simulink model "CartENDI18a"  (R2018a)
settings: Solver=VariableStepAuto  StartTime=0.0  StopTime=Tsim*Nruns  RelTol=1e-3
values from neighbouring files (symbols this model uses):
  delta_t = 0.01    [init.m]
  x0 = [-10; 10; pi/2; 0; 0]    [init.m]    (also in myFindInitState.m = findstates(sys, dataset))
undefined symbols (not defined in the file or in its folder): pars, theta_star
libraries: simulink x1
settings Model: Creator=Osinenko  LastModifiedBy=pavel
settings SFSimCC: SimUseLocalCustomCode=on
settings RTWCC: RTWUseLocalCustomCode=on

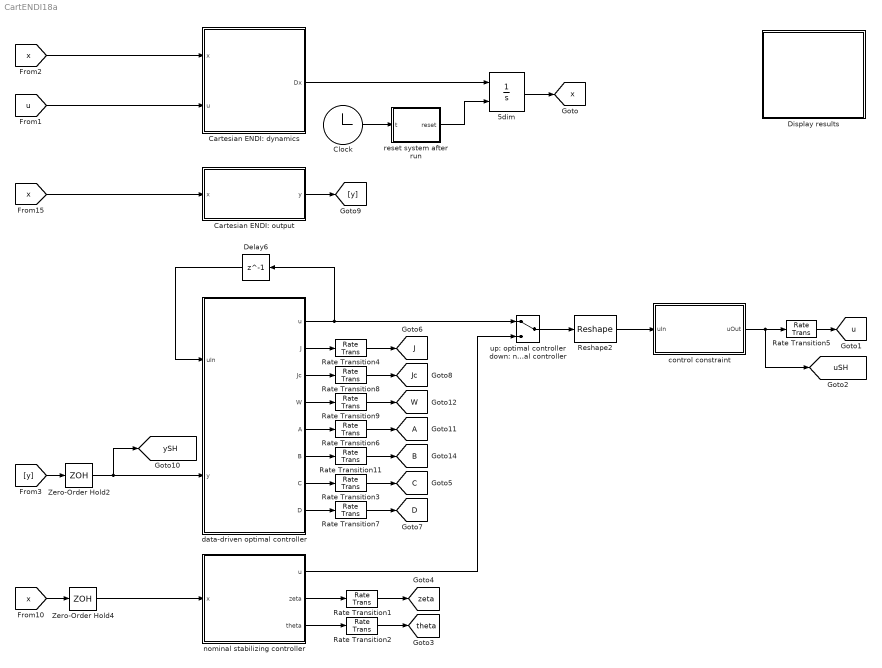
== system CartENDI18a ==
  5dim : Integrator  ExternalReset=rising  InitialCondition=x0
  Cartesian ENDI: dynamics : MATLAB Function  TreatAsAtomicUnit=on
  Cartesian ENDI: output : MATLAB Function  TreatAsAtomicUnit=on
  Clock : Clock
  Delay6 : Delay  DelayLength=1  InitialCondition=0
  Display results : Subsystem
  Rate Transition{1..9,11} (10 alike) : RateTransition
  Reshape2 : Reshape  OutputDimensionality=Customize  OutputDimensions=[pars.dimInput,1]
  Zero-Order Hold2 : ZeroOrderHold  SampleTime=delta_t
  Zero-Order Hold4 : ZeroOrderHold  SampleTime=delta_t
  control constraint : MATLAB Function  TreatAsAtomicUnit=on
  data-driven optimal controller : MATLAB Function  TreatAsAtomicUnit=on
  nominal stabilizing controller : Subsystem
  reset system after run : MATLAB Function  TreatAsAtomicUnit=on
  up: optimal controller down: nominal controller : ManualSwitch
  tag scope: A=global, B=global, C=global, D=global, J=global, Jc=global, W=global, theta=global, u=global, uSH=global, x=global, ySH=global, zeta=global
  wires:
  Cartesian ENDI: dynamics/1(Dx) -> 5dim/1
  5dim/1 -> [x]
  [u] -> Cartesian ENDI: dynamics/2(u)
  [x] -> Cartesian ENDI: dynamics/1(x)
  Rate Transition5/1 -> [u]
  control constraint/1(uOut) -> [uSH], Rate Transition5/1
  Clock/1 -> reset system after run/1(t)
  reset system after run/1(reset) -> 5dim/2
  [x] -> Cartesian ENDI: output/1(x)
  Cartesian ENDI: output/1(y) -> [y]
  nominal stabilizing controller/1(u) -> up: optimal controller down: nominal controller/2
  Rate Transition1/1 -> [zeta]
  Zero-Order Hold4/1 -> nominal stabilizing controller/1(x)
  [x] -> Zero-Order Hold4/1
  nominal stabilizing controller/2(zeta) -> Rate Transition1/1
  nominal stabilizing controller/3(theta) -> Rate Transition2/1
  Rate Transition2/1 -> [theta]
  [y] -> Zero-Order Hold2/1
  Zero-Order Hold2/1 -> [ySH], data-driven optimal controller/2(y)
  Delay6/1 -> data-driven optimal controller/1(uIn)
  data-driven optimal controller/1(u) -> Delay6/1, up: optimal controller down: nominal controller/1
  Rate Transition6/1 -> [A]
  Rate Transition11/1 -> [B]
  data-driven optimal controller/5(A) -> Rate Transition6/1
  data-driven optimal controller/6(B) -> Rate Transition11/1
  Rate Transition3/1 -> [C]
  data-driven optimal controller/7(C) -> Rate Transition3/1
  Rate Transition4/1 -> [J]
  data-driven optimal controller/2(J) -> Rate Transition4/1
  Rate Transition7/1 -> [D]
  data-driven optimal controller/8(D) -> Rate Transition7/1
  Reshape2/1 -> control constraint/1(uIn)
  up: optimal controller down: nominal controller/1 -> Reshape2/1
  Rate Transition8/1 -> [Jc]
  data-driven optimal controller/3(Jc) -> Rate Transition8/1
  Rate Transition9/1 -> [W]
  data-driven optimal controller/4(W) -> Rate Transition9/1

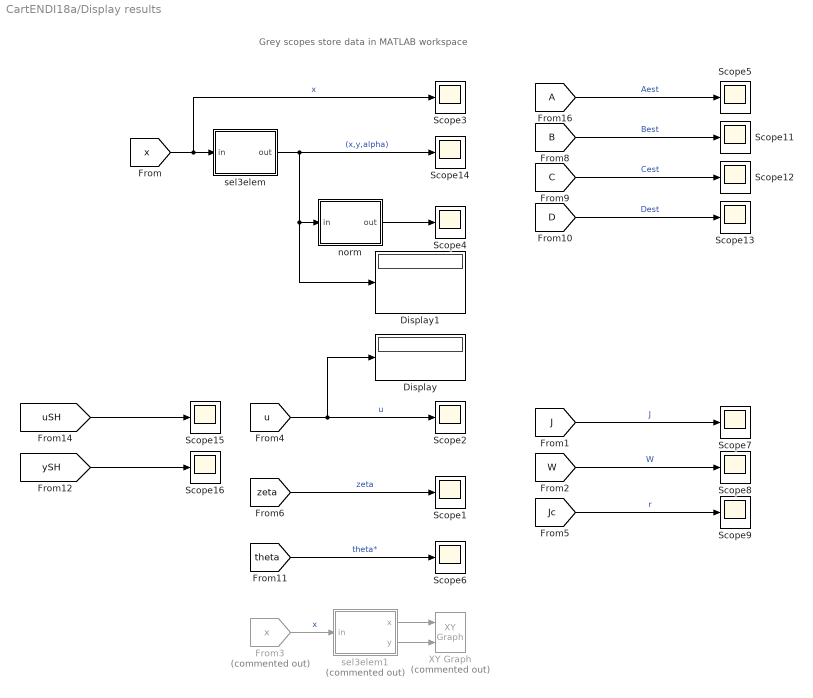
== system CartENDI18a/Display results ==
  note: Grey scopes store data in MATLAB workspace
  Display : Display
  Display1 : Display
  From3 : From  Commented=on  GotoTag=x
  Scope{1..9,11..16} (15 alike) : Scope
  XY Graph : simulink/Sinks/XY Graph  Commented=on  xmin=x_min  xmax=x_max  ymin=y_min  ymax=y_max  st=-1
  norm : MATLAB Function  TreatAsAtomicUnit=on
  sel3elem : MATLAB Function  TreatAsAtomicUnit=on
  sel3elem1 : MATLAB Function  Commented=on  TreatAsAtomicUnit=on
  wires:
  [zeta] -> Scope1/1  "zeta"
  From3/1 -> sel3elem1/1(in)  "x"
  sel3elem1/1(x) -> XY Graph/1
  sel3elem/1(out) -> Scope14/1, Display1/1, norm/1(in)  "(x,y,alpha)"
  [x] -> Scope3/1, sel3elem/1(in)  "x"
  [A] -> Scope5/1  "Aest"
  norm/1(out) -> Scope4/1
  sel3elem1/2(y) -> XY Graph/2
  [u] -> Display/1, Scope2/1  "u"
  [theta] -> Scope6/1  "theta*"
  [J] -> Scope7/1  "J"
  [W] -> Scope8/1  "W"
  [Jc] -> Scope9/1  "r"
  [B] -> Scope11/1  "Best"
  [C] -> Scope12/1  "Cest"
  [D] -> Scope13/1  "Dest"
  [uSH] -> Scope15/1
  [ySH] -> Scope16/1

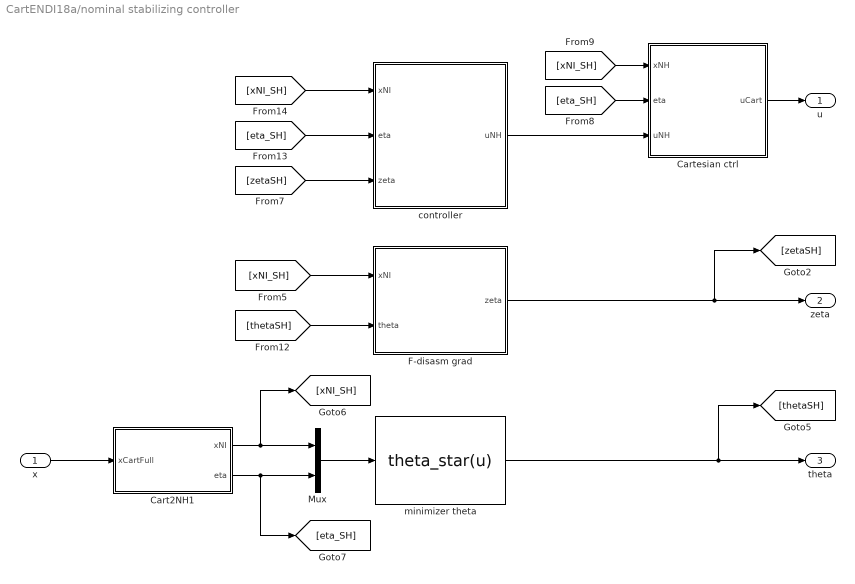
== system CartENDI18a/nominal stabilizing controller ==
  x : Inport
  Cart2NH1 : MATLAB Function  TreatAsAtomicUnit=on
  Cartesian ctrl : MATLAB Function  TreatAsAtomicUnit=on
  F-disasm grad : MATLAB Function  TreatAsAtomicUnit=on
  Mux : Mux  Inputs=2
  controller : MATLAB Function  TreatAsAtomicUnit=on
  minimizer theta : MATLABFcn  MATLABFcn=theta_star(u)
  u : Outport
  zeta : Outport  Port=2
  theta : Outport  Port=3
  wires:
  [xNI_SH] -> Cartesian ctrl/1(xNH)
  minimizer theta/1 -> [thetaSH], theta/1
  F-disasm grad/1(zeta) -> [zetaSH], zeta/1
  [zetaSH] -> controller/3(zeta)
  [eta_SH] -> controller/2(eta)
  Cartesian ctrl/1(uCart) -> u/1
  Cart2NH1/2(eta) -> [eta_SH], Mux/2
  controller/1(uNH) -> Cartesian ctrl/3(uNH)
  [thetaSH] -> F-disasm grad/2(theta)
  Cart2NH1/1(xNI) -> [xNI_SH], Mux/1
  Mux/1 -> minimizer theta/1
  [xNI_SH] -> F-disasm grad/1(xNI)
  [xNI_SH] -> controller/1(xNI)
  x/1 -> Cart2NH1/1(xCartFull)
  [eta_SH] -> Cartesian ctrl/2(eta)

== matlab function CartENDI18a/Display results/norm ==
  data: in input; out output
function out = nrm(in)
%#codegen
%

out = norm(in);

== matlab function CartENDI18a/nominal stabilizing controller/Cart2NH1 ==
  data: xCartFull input; xNI output; eta output
function [xNI, eta] = Cart2NH(xCartFull)
%#codegen
%

xNI = zeros(3, 1);

xc = xCartFull(1);
yc = xCartFull(2);
alpha = xCartFull(3);
v = xCartFull(4);
omega = xCartFull(5);

xNI(1) = alpha;
xNI(2) = xc * cos(alpha) + yc * sin(alpha);
xNI(3) = - 2 * ( yc * cos(alpha) - xc * sin(alpha) ) - alpha * ( xc * cos(alpha) + yc * sin(alpha) );

eta = zeros(2, 1);

eta(1) = omega;
eta(2) = ( yc * cos(alpha) - xc * sin(alpha) ) * omega + v;

== matlab function CartENDI18a/nominal stabilizing controller/controller ==
  data: xNI input; eta input; uNH output; zeta input; pars parameter
function uNH = ctrl(xNI, eta, zeta, pars)
%#codegen
%

uNH = zeros(2, 1);

k = pars.k;

G = zeros(3, 2);

G(:, 1) = [1; 0; xNI(2)];

G(:, 2) = [0; 1; -xNI(1)];

%--------------------------------------------------------------------------
% kappa

kappa = zeros(2, 1);

kappa(1) = - abs( dot( zeta, G(:, 1) ) )^(1/3) * sign( dot( zeta, G(:, 1) ) );
kappa(2) = - abs( dot( zeta, G(:, 2) ) )^(1/3) * sign( dot( zeta, G(:, 2) ) );

%--------------------------------------------------------------------------
% u

z = eta - kappa;

% uNH = G' * zeta - k * z;  <--- for some reason, this doesn't work
uNH = - k * z;

== matlab function CartENDI18a/nominal stabilizing controller/F-disasm grad ==
  data: xNI input; zeta output; theta input
function zeta = disasm_grad_generic(xNI, theta)
%#codegen
%

% x here to mean xNI, the NI-part in nonholonomic form
%
%                                                   3
%                                               |x |
%                   4     4                     | 3|          
%   F(x; theta) = x   +  x   + ----------------------------------------
%                   1     2    
%                               /                                     \ 2
%                              | x cos theta + x sin theta + sqrt|x |  |
%                               \ 1             2                | 3| /
% 
%                                  \_______________  ______________/
%                                                  \/
%                                                 sigma~

sigma_tilde = xNI(1)*cos(theta) + xNI(2)*sin(theta) + sqrt(abs(xNI(3)));

nabla_F = zeros(3,1);

nabla_F(1) = 4*xNI(1)^3 - 2 * abs(xNI(3))^3 * cos(theta)/sigma_tilde^3;

nabla_F(2) = 4*xNI(2)^3 - 2 * abs(xNI(3))^3 * sin(theta)/sigma_tilde^3;

nabla_F(3) = ( 3*xNI(1)*cos(theta) + 3*xNI(2)*sin(theta) + 2*sqrt(abs(xNI(3))) ) * xNI(3)^2 * sign(xNI(3)) / sigma_tilde^3;

zeta = nabla_F;

== matlab function CartENDI18a/Display results/sel3elem1 ==
  data: in input; x output; y output
function [x, y] = sel2elem(in)
%#codegen
%

x = in(1);

y = in(2);

== matlab function CartENDI18a/nominal stabilizing controller/Cartesian ctrl ==
  data: xNH input; eta input; uNH input; uCart output; pars parameter
function uCart = NH2CartCtrl(xNH, eta, uNH, pars)
%#codegen
%

m = pars.m;
I = pars.I;

uCart = zeros(2 ,1);

uCart(1) = m * ( uNH(2) + xNH(2)*eta(1)^2 + 1/2 * ( xNH(1)*xNH(2)*uNH(1) + uNH(1)*xNH(3) ) );
uCart(2) = I * uNH(1);

== matlab function CartENDI18a/Cartesian ENDI: dynamics ==
  data: x input; u input; Dx output; pars parameter
function Dx = sys_rhs(x, u, pars)
%#codegen
%

m = pars.m;
I = pars.I;

Dx = zeros(5, 1);

Dx(1) = x(4) * cos( x(3) );
Dx(2) = x(4) * sin( x(3) );
Dx(3) = x(5);
Dx(4) = 1/m * u(1);
Dx(5) = 1/I * u(2);

% NI only
% Dx = zeros(3, 1);
% 
% Dx(1) = u(1) * cos( x(3) );
% Dx(2) = u(1) * sin( x(3) );
% Dx(3) = u(2);

== matlab function CartENDI18a/reset system after run ==
  data: t input; reset output; pars parameter
function reset = newRun(t, pars)
%#codegen
%

Tsim = pars.Tsim;

if mod(t, Tsim) == 0
    reset = 1;
else
    reset = 0;
end

== matlab function CartENDI18a/Display results/sel3elem ==
  data: in input; out output
function out = sel3elem(in)
%#codegen
%

out = in(1:3);

== matlab function CartENDI18a/Cartesian ENDI: output ==
  data: x input; y output; pars parameter
function y = sys_out(x, pars)
%#codegen
%
% y = x(1:3); % Only position

y = x;      % Position + force/torque sensor

== matlab function CartENDI18a/control constraint ==
  data: uIn input; uOut output; pars parameter
function uOut = ctrlConstraint(uIn, pars)
%#codegen
%

uOut = uIn;

for k = 1:length(uIn)
    if uIn(k) < pars.u_min(k)
        uOut(k) = pars.u_min(k);
    elseif uIn(k) > pars.u_max(k)
        uOut(k) = pars.u_max(k);
    end
end

== matlab function CartENDI18a/data-driven optimal controller ==
  data: uIn input; y input; pars parameter; u output; J output; Jc output; W output; A output; B output; C output; D output
function [u, J, Jc, W, A, B, C, D] = dataDrivOptCtrl(uIn, y, pars)
%#codegen
%dataDrivOptCtrl  Data-driven optimal controller
%
%   Input:
%
%   y               - Measured system output
%   modelPars       - Vector of parameters passed to model-based control (see definition of costFnc below)
%
%   --- Algorithm ---
%
%       Controller seeks to minimize cost
%
%                   N
%           J = sum     r  
%                   1
%
%           where (running cost)
%
%               r = y' * S * y + u' * R * u
%
%
%           and N horizon length
%
%          In RL/ADP, N is interpreted as infinity and so, e.g., in Q-learning, r is substituted for Q-function approximate
%
%          Mode
%             1 - model-predictive control (MPC)
%             2 - MPC with estimated model, a.k.a. adaptive MPC, or AMPC
%             3 - RL/ADP (as stacked Q-learning with horizon N) using true model for prediction
%             4 - RL/ADP (as stacked Q-learning with horizon N) using estimated model for prediction 
%             5 - RL/ADP (as N-step roll-out Q-learning) using true model for prediction
%             6 - RL/ADP (as N-step roll-out Q-learning) using estimated model for prediction 
% 
%             If N = 1, methods are model-free
%
% Critic seeks Q-function approximate as
%
%       Q = W'*phi( y, u )
%
% where W is critic parameters, phi is regressor
%
% W is found by minimizing
%
%                 1       M    2
%           Jc = --   sum     e
%                 2       1
%
%           where (temporal error)
%
%               e = W'*phi( y_prev, u_prev ) - gamma * Wprev'*phi( y_next, u_next ) - r( y_prev, u_prev )
%
%           and M critic stack size
%
%           y's and u's are taken from (parts of) buffers ys, us resp.
%
% Author: P. Osinenko, 2020
% Contact: p.osinenko@gmail.com

%% Initialization: model estimator

dt = pars.delta_t;

% Number of samples (# of delta_t's) between model updates
modelUpdDelay = pars.modelUpdDelay;

% Buffer size for model estimator
Nest = pars.estBufferSize;

modelOrder = pars.modelOrder;

% Number of mode updates
maxModelLearns = pars.modelLearns;

l = pars.dimInput;
p = length(y);

if isrow(uIn)
    uIn = uIn';
end

if isrow(y)
    y = y';
end

persistent us;
if isempty(us)
    us = zeros(l, Nest);
end

persistent ys;
if isempty(ys)
    ys = zeros(p, Nest);
end

persistent timer;
if isempty(timer)
    timer = 1;
end

persistent myA;
if isempty(myA)
    % myA = zeros(modelOrder);
    myA = pars.Aest0;
end
persistent myB;
if isempty(myB)
    % myB = zeros(modelOrder, l);
    myB = pars.Best0;
end
persistent myC;
if isempty(myC)
    % myC = zeros(p, modelOrder);
    myC = pars.Cest0;
end
persistent myD;
if isempty(myD)
    myD = pars.Dest0;
end
% persistent my_x0set;
% if isempty(my_x0set)
%     my_x0set = zeros(modelOrder, 1);
% end
persistent modelLearns;
if isempty(modelLearns)
    modelLearns = 0;
end

coder.extrinsic('mySSest');
coder.extrinsic('myFindInitState');

%% Initialization: actor

% Horizon length for controller
Nctrl = pars.ctrlStackSize;

modelPars = [pars.m pars.I];

S = pars.rcostS;
R = pars.rcostR;

u_min = pars.u_min;
u_max = pars.u_max;

u_init = u_min/2;
Uinit = repmat(u_init, 1, Nctrl);  

mode = pars.optCtrlMode;

coder.extrinsic('optCtrl');

%% Initialization: critic

% Number of samples (# of delta_t's) between critic updates
criticUpdDelay = pars.criticUpdDelay;

% Number of critic updates
maxCriticLearns = pars.criticLearns;

persistent criticLearns;
if isempty(criticLearns)
    criticLearns = 0;
end

% Critic stack size
Ncrit = pars.criticStackSize; 

gamma = pars.gamma;

W = pars.W0;

persistent Wprev
if isempty(Wprev)
    Wprev = W;
end

Wmin = pars.Wmin;
Wmax = pars.Wmax;

Winit = Wprev;

coder.extrinsic('critic');

critStruct = pars.critStruct;

%% Model estimator

% Update data buffers
us = pushCol(us, uIn);
ys = pushCol(ys, y);

% Update model when buffer is full and modelUpdDelay is elapsed
if (timer >= Nest) && (mod(timer, modelUpdDelay) == 0) && ( Nctrl > 1 ) && ( (mode == 2) || (mode == 4) || (mode == 6) ) && (modelLearns < maxModelLearns)
    [myA, myB, myC, myD] = mySSest(ys, us, dt, modelOrder);
%     [myA, myB, myC, myD] = mySSest(ys, us, dt, modelOrder, myA, myB, myC, myD);   % < -- using previous estimate as initial guess
    modelLearns = modelLearns + 1;
end

A = myA;
B = myB;
C = myC;
D = myD;
% x0est = my_x0set;
% x0est = myFindInitState(A, B, C, D, us, ys, dt);
x0est = myFindInitState(A, B, C, D, u_init, y, dt);

%% Critic

Jc = 0;

% Update critic when criticUpdDelay is elapsed
if (mod(timer, criticUpdDelay) == 0) && ( (mode == 3) || (mode == 4) || (mode == 5) || (mode == 6) ) && (criticLearns < maxCriticLearns)
    [W, Jc] = critic(Wprev, Winit, us(:,end-Ncrit+1:end), ys(:,end-Ncrit+1:end), S, R, Ncrit, gamma, Wmin, Wmax, critStruct);
    Wprev = W;
    criticLearns = criticLearns + 1;
else
    W = Wprev;
end


%% Controller

u = zeros(l, 1);
J = 0;

if timer < Nest
    u = pars.probNoisePow*randn(l, 1);
else
    [u, J] = optCtrl(y, Uinit, S, R, Nctrl, W, A, B, C, D, x0est, mode, u_min, u_max, dt, modelPars, critStruct);
end

if pars.isProbNoise
    u = u + pars.probNoisePow*randn(l, 1);
end

timer = timer + 1;

function Y = pushCol(X, v)
% Push column vector v to the right of matrix X

% Y = [X(:, 2) X(:, 3) ... X(:, N) v]

[n, m]  = size(X);
Y       = zeros(n, m);

Y(:, m)  = v;

for II = 1:m-1
    Y(:, II) = X(:, II+1);
end
